simulink model "SlidControlSignSim"  (R2018a)
settings: Solver=VariableStepAuto  StartTime=0.0  StopTime=20  RelTol=1e-3
values from neighbouring files (symbols this model uses):
  A = [a 0;1 0]    [SlidingControl.m]
  B = [b;0]    [SlidingControl.m]
  D = [1;0]    [SlidingControl.m]
  dmax = 0.9    [SlidingControl.m]
  Mu = 0.5    [SlidingControl.m]
  surf_C = [c1;c2]    [SlidingControl.m]
settings Model: Creator=ageng  LastModifiedBy=ageng
settings SolverCC: ZeroCrossAlgorithm=Adaptive
settings DebuggingCC: MaxConsecutiveZCsMsg=none

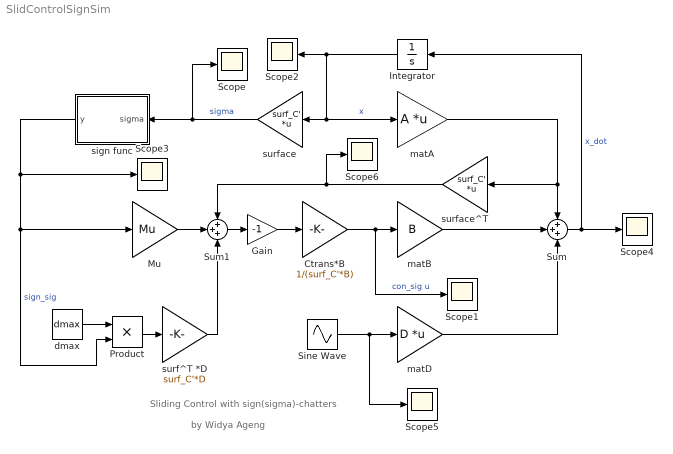
== system SlidControlSignSim ==
  note: by Widya Ageng
  note: Sliding Control with sign(sigma)-chatters
  "Ctrans*B " : Gain  Gain=1/(surf_C'*B)
  Gain : Gain  Gain=-1
  Integrator : Integrator  InitialCondition=[1;1]
  Mu : Gain  Gain=Mu
  Product : Product
  Scope{,1..6} (7 alike) : Scope
  Sine Wave : Sin  Amplitude=0  Frequency=628  SampleTime=0.0001
  Sum : Sum  Inputs=+++
  Sum1 : Sum  Inputs=+++
  dmax : Constant  Value=dmax  SampleTime=0.0001
  matA : Gain  Gain=A  Multiplication=Matrix(K*u) (u vector)
  matB : Gain  Gain=B
  matD : Gain  Gain=D  Multiplication=Matrix(K*u) (u vector)
  sign func : MATLAB Function  TreatAsAtomicUnit=on
  surf^T *D : Gain  Gain=surf_C'*D
  "surface " : Gain  Gain=surf_C'  Multiplication=Matrix(K*u) (u vector)
  surface^T : Gain  Gain=surf_C'  Multiplication=Matrix(K*u) (u vector)
  wires:
  Integrator/1 -> Scope2/1, "surface "/1, matA/1  "x"
  matA/1 -> surface^T/1, Sum/1
  matB/1 -> Sum/2
  Sum/1 -> Scope4/1, Integrator/1  "x_dot"
  surface^T/1 -> Scope6/1, Sum1/1
  "surface "/1 -> sign func/1(sigma), Scope/1  "sigma"
  Mu/1 -> Sum1/2
  sign func/1(y) -> Scope3/1, Product/2, Mu/1  "sign_sig"
  Sum1/1 -> Gain/1
  Gain/1 -> "Ctrans*B "/1
  "Ctrans*B "/1 -> Scope1/1, matB/1  "con_sig u"
  Sine Wave/1 -> Scope5/1, matD/1
  surf^T *D/1 -> Sum1/3
  matD/1 -> Sum/3
  dmax/1 -> Product/1
  Product/1 -> surf^T *D/1

== matlab function SlidControlSignSim/sign func ==
  data: sigma input; y output
function y = fcn(sigma)

epsilon = 0.01;

if sigma>0
    out = 1;
else
    out = -1;
end

y = out;
